simulink model "MainSimulink"  (R2020a)
settings: Solver=VariableStepAuto  StartTime=0.0  StopTime=20.0  RelTol=1e-3
values from neighbouring files (symbols this model uses):
  a = 1    [TransferFunc.m]
  c = 1    [TransferFunc.m]
  d = 2    [TransferFunc.m]
settings Model: Creator=Alexandru Olteanu  LastModifiedBy=Alexandru Olteanu

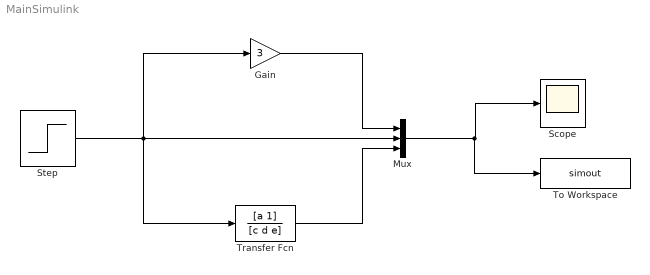
== system MainSimulink ==
  Gain : Gain  Gain=3
  Mux : Mux  Inputs=3
  Scope : Scope
  Step : Step  Time=5  Before=2  After=4  SampleTime=0
  To Workspace : ToWorkspace  VariableName=simout  SaveFormat=Timeseries  SampleTime=-1
  Transfer Fcn : TransferFcn  Numerator=[a 1]  Denominator=[c d e]
  wires:
  Step/1 -> Mux/2, Gain/1, Transfer Fcn/1
  Transfer Fcn/1 -> Mux/3
  Gain/1 -> Mux/1
  Mux/1 -> To Workspace/1, Scope/1
